simulink model "solar_heating_source_20241116"  (R2024a)
settings: Solver=VariableStepAuto  StartTime=0.0  StopTime=10.0  RelTol=1e-3
libraries: fl_lib x10, nesl_utility x3
settings Model: Creator=fanzh  LastModifiedBy=fanzh

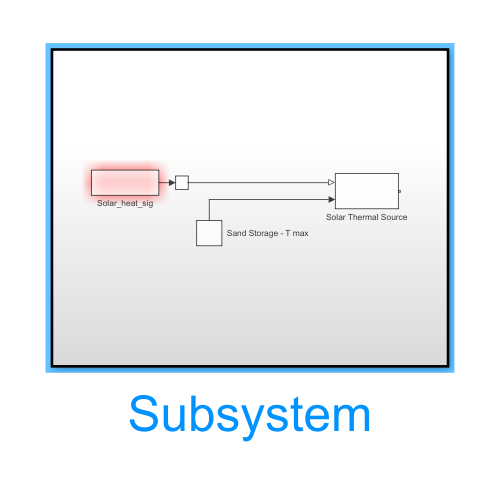
[thumbnail: Simulink's stored preview of the top-level diagram]
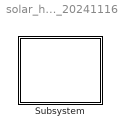
== system solar_heating_source_20241116 ==
  Subsystem : Subsystem

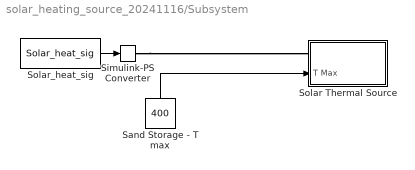
== system solar_heating_source_20241116/Subsystem ==
  Sand Storage - T max : Constant  Value=400
  Simulink-PS Converter : nesl_utility/Simulink-PS Converter  PhysicalDomain=network_engine_domain  SubClassName=ps_input  LeftPortType=input  RightPortType=output  PseudoPeriodic=off  Frequencies=[]  NoiseDistribution=none  NoiseParameters=[]  Unit=1  AffineConversion=off  FilteringAndDerivatives=provide  SimscapeFilterOrder=1  InputFilterTimeConstant=0.001  UdotUserProvided=0
  Solar Thermal Source : Subsystem
      settings: PortSchema="{\"entries\":[{\"content\":{\"sides\":[{\"content\":{\"connectorIds\":[\"LConn1\",\"In1\"]},\"type\":\"ConnectorPlacement.EquallySpacedRectSide\",\"uuid\":\"f69a8d61-d6b7-4c5f-bee5-6777f6738a93\"},{\"content\":{\"connectorIds\":[\"RConn1\"],\"side\":\"RIGHT\"},\"type\":\"ConnectorPlacement.EquallySpacedRectSide\",\"uuid\":\"2abf6aad-3ae7-4bac-8cd7-a5726210c2fc\"},{\"content\":{\"side\":\"TOP\"},\"type\":\"ConnectorPlacement.EquallySpacedRectSide\",\"uuid\":\"e643bfa7-5cdc-456c-a6d6-e9bc07f127d5\"}]},\"type\":\"ConnectorPlacement.EquallySpacedConnector\",\"uuid\":\"a763efd1-4c7b-49c2-88ea-f9b1ada0c58b\"}],\"packageUris\":[\"http://schema.mathworks.com/mf0/Connector/R2020b\"],\"version\":\"1.0\"}"
  Solar_heat_sig : FromWorkspace  VariableName=Solar_heat_sig  OutDataTypeStr=boolean  SampleTime=10  Interpolate=off  ZeroCross=off  OutputAfterFinalValue=Holding final value
  wires:
  Solar_heat_sig/1 -> Simulink-PS Converter/1
  Sand Storage - T max/1 -> Solar Thermal Source/1(T Max)
  connections:
  Simulink-PS Converter/RConn1 -- Solar Thermal Source/LConn1

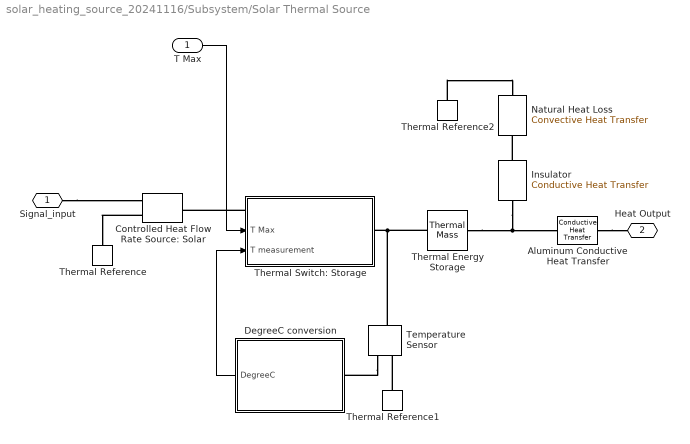
== system solar_heating_source_20241116/Subsystem/Solar Thermal Source ==
  T Max : Inport
  Aluminum Conductive Heat Transfer : fl_lib/Thermal/Thermal Elements/Conductive Heat Transfer  thermal_type=foundation.enum.ConstantVariableTabulated.Constant  wall_geometry=foundation.enum.ConductionWallGeometry.Planar  area=4e-4 m^2  thickness=0.1 m  d_in=0.05 m  d_out=0.1 m  L=1 m  th_cond_min=10 W/(K*m)  th_cond=237 W/(K*m)  th_cond_TLU=[413, 401, 392, 383, 371, 357, 342] W/(K*m)  temp_TLU=[200, 273, 400, 600, 800, 1000, 1200] K  T_specify=off  T_priority=None  T=0 K  T_nominal_specify=off  T_nominal_value=1  T_nominal_unit=K  Q_specify=off  Q_priority=None  Q=0 W  Q_nominal_specify=off  Q_nominal_value=1  Q_nominal_unit=W
  Controlled Heat Flow Rate Source: Solar : fl_lib/Thermal/Thermal Sources/Controlled Heat Flow Rate Source
  DegreeC conversion : Subsystem
  Insulator : fl_lib/Thermal/Thermal Elements/Conductive Heat Transfer  thermal_type=foundation.enum.ConstantVariableTabulated.Constant  wall_geometry=foundation.enum.ConductionWallGeometry.Planar  area=1e-3 m^2  thickness=0.1 m  d_in=0.05 m  d_out=0.1 m  L=1 m  th_cond_min=10 W/(K*m)  th_cond=0.1 W/(K*m)  th_cond_TLU=[413, 401, 392, 383, 371, 357, 342] W/(K*m)  temp_TLU=[200, 273, 400, 600, 800, 1000, 1200] K  T_specify=off  T_priority=None  T=0 K  T_nominal_specify=off  T_nominal_value=1  T_nominal_unit=K  Q_specify=off  Q_priority=None  Q=0 W  Q_nominal_specify=off  Q_nominal_value=1  Q_nominal_unit=W
  Natural Heat Loss : fl_lib/Thermal/Thermal Elements/Convective Heat Transfer  thermal_type=foundation.enum.constant_variable.constant  area=1e-3 m^2  heat_tr_coeff=10 W/(K*m^2)  min_heat_tr_coeff=1e-3 W/(K*m^2)  T_specify=off  T_priority=None  T=0 K  T_nominal_specify=off  T_nominal_value=1  T_nominal_unit=K  Q_specify=off  Q_priority=None  Q=0 W  Q_nominal_specify=off  Q_nominal_value=1  Q_nominal_unit=W
  Temperature Sensor : fl_lib/Thermal/Thermal Sensors/Temperature Sensor  temperature_measure=foundation.enum.MeasurementReference.difference
  Thermal Energy Storage : fl_lib/Thermal/Thermal Elements/Thermal Mass  mass_type=foundation.enum.constant_variable.constant  mass=10 kg  sp_heat=840 J/(K*kg)  mass_min=1e-6 kg  num_ports=foundation.enum.numPorts2.two  m_specify=off  m_priority=High  m=1 kg  m_nominal_specify=off  m_nominal_value=1  m_nominal_unit=kg  T_specify=off  T_priority=High  T=300 K  T_nominal_specify=off  T_nominal_value=1  T_nominal_unit=K  Q_specify=off  Q_priority=None  Q=0 W  Q_nominal_specify=off  Q_nominal_value=1  Q_nominal_unit=W
      settings: InternalSimscapePortConfiguration="{\"Bottom\":[],\"Left\":[{\"id\":\"M\",\"label\":\"\",\"type\":\"foundation.thermal.thermal\"}],\"Right\":[{\"id\":\"N\",\"label\":\"\",\"type\":\"foundation.thermal.thermal\"}],\"Top\":[]}"
  Thermal Reference : fl_lib/Thermal/Thermal Elements/Thermal Reference
  Thermal Reference1 : fl_lib/Thermal/Thermal Elements/Thermal Reference
  Thermal Reference2 : fl_lib/Thermal/Thermal Elements/Thermal Reference
  Thermal Switch: Storage : Subsystem
      settings: PortSchema="{\"entries\":[{\"content\":{\"sides\":[{\"content\":{\"connectorIds\":[\"LConn1\",\"In1\",\"In2\"]},\"type\":\"ConnectorPlacement.EquallySpacedRectSide\",\"uuid\":\"eab90983-c678-4d00-88f4-d7eb0332fabb\"},{\"content\":{\"connectorIds\":[\"RConn1\"],\"side\":\"RIGHT\"},\"type\":\"ConnectorPlacement.EquallySpacedRectSide\",\"uuid\":\"4911cae5-9d9f-472e-86e2-92bac9c7b6a6\"},{\"content\":{\"side\":\"TOP\"},\"type\":\"ConnectorPlacement.EquallySpacedRectSide\",\"uuid\":\"e0869e9b-2d53-4209-96a5-637bff90aadc\"}]},\"type\":\"ConnectorPlacement.EquallySpacedConnector\",\"uuid\":\"c03f20a9-89c5-4bd4-ab09-4122887b8deb\"}],\"packageUris\":[\"http://schema.mathworks.com/mf0/Connector/R2020b\"],\"version\":\"1.0\"}"
  Signal_input : PMIOPort  Side=Left
  Heat Output : PMIOPort  Port=2  Side=Right
  wires:
  T Max/1 -> Thermal Switch: Storage/1(T Max)
  DegreeC conversion/1(DegreeC) -> Thermal Switch: Storage/2(T measurement)
  connections:
  Thermal Reference2/LConn1 -- Natural Heat Loss/RConn1
  Thermal Energy Storage/LConn1 -- Insulator/LConn1 -- Aluminum Conductive Heat Transfer/LConn1
  Thermal Energy Storage/RConn1 -- Temperature Sensor/LConn1 -- Thermal Switch: Storage/RConn1
  Temperature Sensor/RConn2 -- DegreeC conversion/LConn1
  Thermal Reference1/LConn1 -- Temperature Sensor/RConn1
  Insulator/RConn1 -- Natural Heat Loss/LConn1
  Thermal Switch: Storage/LConn1 -- Controlled Heat Flow Rate Source: Solar/LConn1
  Controlled Heat Flow Rate Source: Solar/RConn2 -- Thermal Reference/LConn1
  Signal_input/RConn1 -- Controlled Heat Flow Rate Source: Solar/RConn1
  Aluminum Conductive Heat Transfer/RConn1 -- Heat Output/RConn1

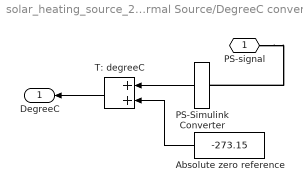
== system solar_heating_source_20241116/Subsystem/Solar Thermal Source/DegreeC conversion ==
  Absolute zero reference : Constant  Value=-273.15
  PS-Simulink Converter : nesl_utility/PS-Simulink Converter  PhysicalDomain=network_engine_domain  SubClassName=ps_output  LeftPortType=input  RightPortType=output  PseudoPeriodic=off  Frequencies=[]  VectorFormat=inherit  Unit=inherit  AffineConversion=off
  T: degreeC : Sum
  PS-signal : PMIOPort  Side=Left
  DegreeC : Outport
  wires:
  Absolute zero reference/1 -> T: degreeC/2
  PS-Simulink Converter/1 -> T: degreeC/1
  T: degreeC/1 -> DegreeC/1
  connections:
  PS-signal/RConn1 -- PS-Simulink Converter/LConn1

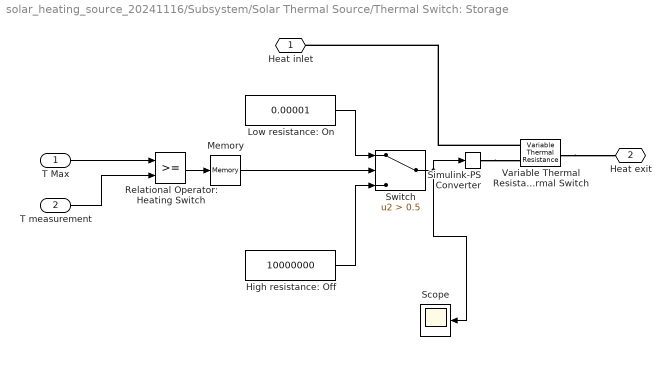
== system solar_heating_source_20241116/Subsystem/Solar Thermal Source/Thermal Switch: Storage ==
  T Max : Inport
  T measurement : Inport  Port=2
  High resistance: Off : Constant  Value=10000000
  Low resistance: On : Constant  Value=0.00001
  Memory : Memory
  Relational Operator: Heating Switch : RelationalOperator  OutDataTypeStr=boolean  RndMeth=Simplest  InputSameDT=off
  Scope : Scope
  Simulink-PS Converter : nesl_utility/Simulink-PS Converter  PhysicalDomain=network_engine_domain  SubClassName=ps_input  LeftPortType=input  RightPortType=output  PseudoPeriodic=off  Frequencies=[]  NoiseDistribution=none  NoiseParameters=[]  Unit=1  AffineConversion=off  FilteringAndDerivatives=provide  SimscapeFilterOrder=1  InputFilterTimeConstant=0.001  UdotUserProvided=0
  Switch : Switch  Criteria=u2 > Threshold  Threshold=0.5  SaturateOnIntegerOverflow=off  InputSameDT=off
  Variable Thermal Resistance: Thermal Switch : fl_lib/Thermal/Thermal Elements/Variable Thermal Resistance  R_min=0 K/W  T_specify=off  T_priority=None  T=0 K  T_nominal_specify=off  T_nominal_value=1  T_nominal_unit=K  Q_specify=off  Q_priority=None  Q=0 W  Q_nominal_specify=off  Q_nominal_value=1  Q_nominal_unit=W
      settings: InternalSimscapePortConfiguration="{\"Bottom\":[],\"Left\":[{\"id\":\"A\",\"label\":\"A\",\"type\":\"foundation.thermal.thermal\"},{\"id\":\"R\",\"label\":\"R\",\"type\":\"input\"}],\"Right\":[{\"id\":\"B\",\"label\":\"B\",\"type\":\"foundation.thermal.thermal\"}],\"Top\":[]}"
  Heat inlet : PMIOPort  Side=Left
  Heat exit : PMIOPort  Port=2  Side=Right
  wires:
  Relational Operator: Heating Switch/1 -> Memory/1
  T measurement/1 -> Relational Operator: Heating Switch/2
  High resistance: Off/1 -> Switch/3
  Switch/1 -> Scope/1, Simulink-PS Converter/1
  T Max/1 -> Relational Operator: Heating Switch/1
  Low resistance: On/1 -> Switch/1
  Memory/1 -> Switch/2
  connections:
  Simulink-PS Converter/RConn1 -- Variable Thermal Resistance: Thermal Switch/LConn2
  Variable Thermal Resistance: Thermal Switch/LConn1 -- Heat inlet/RConn1
  Variable Thermal Resistance: Thermal Switch/RConn1 -- Heat exit/RConn1
